simulink model "SpeedToFreq"  (R2023a)
settings: Solver=VariableStepAuto  StartTime=0.0  StopTime=10.0  RelTol=1e-3
settings Model: Creator=ela19kfs  LastModifiedBy=ela19kfs

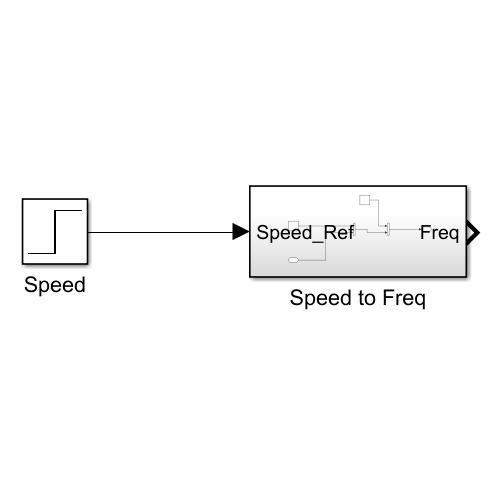
[thumbnail: Simulink's stored preview of the top-level diagram]
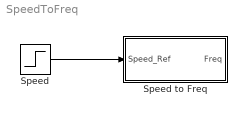
== system SpeedToFreq ==
  Speed : Step  SampleTime=0
  Speed to Freq : Subsystem
  wires:
  Speed/1 -> Speed to Freq/1(Speed_Ref)

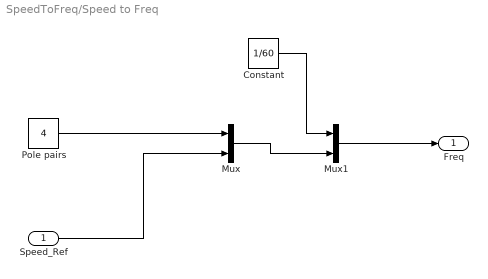
== system SpeedToFreq/Speed to Freq ==
  Speed_Ref : Inport
  Constant : Constant  Value=1/60
  Mux : Mux  Inputs=2
      settings: DisplayOption=signals
  Mux1 : Mux  Inputs=2
  Pole pairs : Constant  Value=4
  Freq : Outport
  wires:
  Speed_Ref/1 -> Mux/2
  Pole pairs/1 -> Mux/1
  Constant/1 -> Mux1/1
  Mux/1 -> Mux1/2
  Mux1/1 -> Freq/1
